simulink model "untitled"  (R2022a)
settings: Solver=FixedStepAuto  StartTime=0.0  StopTime=10.0  RelTol=1e-3  EnableMultiTasking=on
settings Model: ExtModeTrigDuration=2  Creator=sa.salehi  LastModifiedBy=Asus
settings OptimizationCC: EnhancedBackFolding=on  PassReuseOutputArgsAs=Individual arguments  ZeroExternalMemoryAtStartup=off  ZeroInternalMemoryAtStartup=off  MaxStackSize=64  OptimizeBlockOrder=speed  DifferentSizesBufferReuse=on  OptimizationCustomize=off  EfficientTunableParamExpr=on
settings DebuggingCC: ParameterTunabilityLossMsg=error
settings HardwareCC: ProdBitPerInt=16  ProdBitPerPointer=16  ProdBitPerSizeT=16  ProdBitPerPtrDiffT=16  ProdLargestAtomicFloat=None  ProdWordSize=8  ProdHWDeviceType=Atmel->AVR
settings ModelReferenceCC: EnableRefExpFcnMdlSchedulingChecks=off
settings SFSimCC: MATLABDynamicMemAlloc=off
settings RTWCC: SystemTargetFile=ert.tlc  HardwareBoard=Arduino Uno  GenCodeOnly=on  TemplateMakefile=ert_default_tmf  GenerateReport=on  Toolchain=Arduino AVR  BuildConfiguration=Faster Runs  LaunchReport=on
settings CodeAppCC: ForceParamTrailComments=on  IgnoreCustomStorageClasses=off  OperatorAnnotations=on  SimulinkDataObjDesc=on  SFDataObjDesc=on  InsertBlockDesc=on
settings ERTTargetCC: SupportContinuousTime=on  SupportVariableSizeSignals=on  ExtModeTransport=3  ExtModeStaticAlloc=on  ExtModeStaticAllocSize=250  ExtModeMexFile=ext_xcp  ExtModeIntrfLevel=Level2 - Open

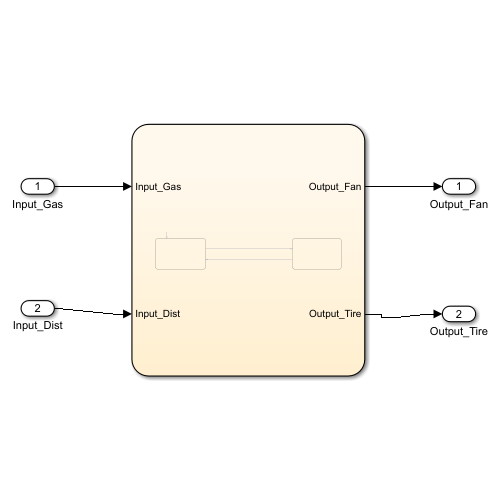
[thumbnail: Simulink's stored preview of the top-level diagram]
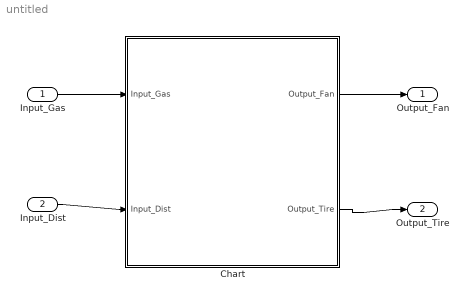
== system untitled ==
  Input_Gas : Inport
  Input_Dist : Inport  Port=2
  Chart : Stateflow chart  TreatAsAtomicUnit=on
  Output_Fan : Outport
  Output_Tire : Outport  Port=2
  wires:
  Input_Gas/1 -> Chart/1(Input_Gas)
  Input_Dist/1 -> Chart/2(Input_Dist)
  Chart/2(Output_Tire) -> Output_Tire/1
  Chart/1(Output_Fan) -> Output_Fan/1

== stateflow chart untitled/Chart ==
  state forward
  state backward
  (default) -> forward
  forward -> backward : [Input_Gas >52 || Input_Dist < 1.02]{Output_Tire=0; Output_Fan=0;}
  backward -> forward : [Input_Gas <48 && Input_Dist > 0.98]{Output_Tire=1; Output_Fan=1;}
  data: Output_Fan output =1; Input_Gas input; Input_Dist input; Output_Tire output =1
